simulink model "ModelEquationsDOF4"  (R2022b)
settings: Solver=ode4  StartTime=0.0  StopTime=100  FixedStep=10^-3  RelTol=1e-3
values from neighbouring files (symbols this model uses):
  C1 = 310    [ModelFixedParamDOF4.m]
  C2 = 200    [ModelFixedParamDOF4.m]
  C3 = 9091    [ModelFixedParamDOF4.m]
  C4 = 330    [ModelFixedParamDOF4.m]
  C5 = 2475    [ModelFixedParamDOF4.m]
  Cs = 74518    [OptimizedParamDOF3.m]    (also in OptimizedParamDOF4.m = 900)
  Cse = 150    [ModelFixedParamDOF4.m]
  Ct = 850    [ModelFixedParamDOF3.m]    (also in ModelFixedParamDOF4.m)
  K1 = 166990    [ModelFixedParamDOF4.m]
  K2 = 10000    [ModelFixedParamDOF4.m]
  K3 = 144000    [ModelFixedParamDOF4.m]
  K4 = 20000    [ModelFixedParamDOF4.m]
  K5 = 49340    [ModelFixedParamDOF4.m]
  Ks = 106826    [OptimizedParamDOF3.m]    (also in OptimizedParamDOF4.m = 10039)
  Kse = 15000    [ModelFixedParamDOF4.m]
  Kt = 150000    [ModelFixedParamDOF3.m]    (also in ModelFixedParamDOF4.m)
  m1 = 417    [ModelFixedParamDOF4.m]    (also in ModelFixedParamDOF5.m = 40)
  m2 = 15    [ModelFixedParamDOF4.m]    (also in ModelFixedParamDOF5.m = 35.5)
  m3 = 55    [ModelFixedParamDOF4.m]
  m4 = 36    [ModelFixedParamDOF4.m]
  mb = 250    [ModelFixedParamDOF4.m]
  mse = 35    [ModelFixedParamDOF4.m]
  mw = 25    [ModelFixedParamDOF4.m]
  road_front_wheel = M.'    [LoadRoadScript.m]
settings Model: Creator=Ade  LastModifiedBy=andre
settings SolverCC: AlgebraicLoopSolver=TrustRegion
settings DataIOCC: ReturnWorkspaceOutputs=off
settings DebuggingCC: UnconnectedInputMsg=warning  UnconnectedOutputMsg=warning  UnconnectedLineMsg=warning  SFMachineParentedDataDiag=warning  ArithmeticOperatorsInVariantConditions=warning
settings ModelReferenceCC: EnableRefExpFcnMdlSchedulingChecks=on
settings SFSimCC: SimUseLocalCustomCode=off  CustomCodeUndefinedFunction=UseInterfaceOnly
settings RTWCC: RTWUseLocalCustomCode=off  DLArmComputeVersion=19.05

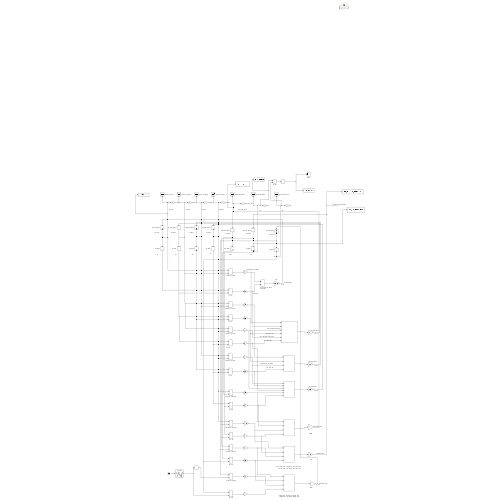
[thumbnail: Simulink's stored preview of the top-level diagram]
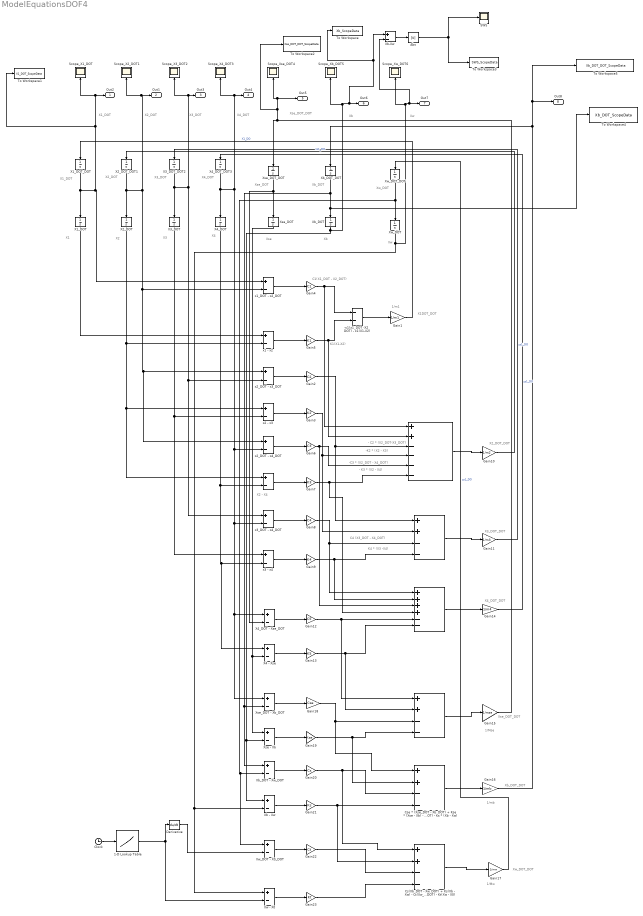
== system ModelEquationsDOF4 ==
  note: 1/Mw
  note: X4_DOT_DOT
  note: X3_DOT_DOT
  note: C4 (X3_DOT - X4_DOT)
  note: K4 * (X3 -X4)
  note: X2 - X4
  note: X2_DOT_DOT
  note: - K3 * (X2 - X4)
  note: -C3 * (X2_DOT - X4_DOT)
  note: K1(X1-X2)
  note: C1(X1_DOT - X2_DOT)
  note: 1/m1
  note: X3
  note: X4
  note: X2
  note: X1_DOT
  note: X1DOT_DOT
  note: X2_DOT
  note: X1
  note: X3_DOT
  note: X4_DOT
  note: -K2 * (X2 - X3)
  note: - C2 * (X2_DOT-X3_DOT)
  note: Xse_DOT
  note: Xse
  note: Xb
  note: Xb_DOT
  note: Xw
  note: Xw_DOT
  note: Xse_DOT_DOT
  note: Xw_DOT_DOT
  note: Xb_DOT_DOT
  note: 1/mb
  note: 1/Mse
  note: X1_DOT
  note: X2_DOT
  note: X3_DOT
  note: X4_DOT
  note: Xse_DOT_DOT
  note: Xb
  note: Xw
  " " : Sum  Inputs=+-
  "      " : Sum  Inputs=++----
  " " : Sum  Inputs=++--
  " " : Sum  Inputs=++++--
  " " : Sum  Inputs=++--
  " Cs(Xb_DOT - Xw_DOT) + Ks(Xb - Xw) - Ct(Xw_DOT - X0_DOT) - Kt(Xw - X0)" : Sum  Inputs=++--
  " Cse * (Xse_DOT - Xb_DOT) + Kse * (Xse - Xb) - Cs * (Xb_DOT - Xw_DOT) - Ks * (Xb - Xw)" : Sum  Inputs=++--
  "                    -c1(x1_DOT -X2_DOT) - k1(X1-X2)" : Sum  Inputs=--
  1-D Lookup Table : Lookup_n-D  NumberOfTableDimensions=1  LookupTableObject=road_front_wheel  BreakpointsForDimension1=[1:100]  Table=road_front_wheel  InternalRulePriority=Speed  RndMeth=Simplest
  Abs : Abs  SaturateOnIntegerOverflow=off
  Clock : Clock
  Derivative : Derivative
  Gain1 : Gain  Gain=1/m1
  Gain10 : Gain  Gain=1/m2
  Gain11 : Gain  Gain=1/m3
  Gain12 : Gain  Gain=C5
  Gain13 : Gain  Gain=K5
  Gain14 : Gain  Gain=1/m4
  Gain15 : Gain  Gain=1/mse
  Gain16 : Gain  Gain=1/mb
  Gain17 : Gain  Gain=1/mw
  Gain18 : Gain  Gain=Cse
  Gain19 : Gain  Gain=Kse
  Gain2 : Gain  Gain=C2
  Gain20 : Gain  Gain=Cs
  Gain21 : Gain  Gain=Ks
  Gain22 : Gain  Gain=Ct
  Gain23 : Gain  Gain=Kt
  Gain3 : Gain  Gain=K2
  Gain4 : Gain  Gain=C1
  Gain5 : Gain  Gain=K1
  Gain6 : Gain  Gain=C3
  Gain7 : Gain  Gain=K3
  Gain8 : Gain  Gain=C4
  Gain9 : Gain  Gain=K4
  SWS : Scope
  Scope_X1_DOT : Scope
  Scope_X2_DOT1 : Scope
  Scope_X3_DOT2 : Scope
  Scope_X4_DOT3 : Scope
  Scope_Xb_DOT5 : Scope
  Scope_Xse_DOT4 : Scope
  Scope_Xw_DOT6 : Scope
  To Workspace : ToWorkspace  VariableName=Xb_ScopeData  SaveFormat=Structure With Time  SampleTime=-1
  To Workspace1 : ToWorkspace  VariableName=X1_DOT_ScopeData  SaveFormat=Structure With Time  SampleTime=-1
  To Workspace2 : ToWorkspace  VariableName=Xse_DOT_DOT_ScopeData  SaveFormat=Structure With Time  SampleTime=-1
  To Workspace3 : ToWorkspace  VariableName=SWS_ScopeData  SaveFormat=Structure With Time  SampleTime=-1
  To Workspace4 : ToWorkspace  VariableName=Xb_DOT_ScopeData  SaveFormat=Structure With Time  SampleTime=-1
  To Workspace5 : ToWorkspace  VariableName=Xb_DOT_DOT_ScopeData  SaveFormat=Structure With Time  SampleTime=-1
  X1_DOT : Integrator
  X1_DOT_DOT : Integrator
  X2_DOT : Integrator
  X2_DOT_DOT1 : Integrator
  X3_DOT : Integrator
  X3_DOT_DOT2 : Integrator
  X4 - Xse : Sum  Inputs=+-
  X4_DOT : Integrator
  X4_DOT - Xse_DOT : Sum  Inputs=+-
  X4_DOT_DOT3 : Integrator
  Xb - Xw : Sum  Inputs=+-
  Xb-Xw : Sum  Inputs=+-
  Xb_DOT : Integrator
  Xb_DOT - Xw_DOT : Sum  Inputs=+-
  Xb_DOT_DOT : Integrator
  Xse - Xb : Sum  Inputs=+-
  Xse_DOT : Integrator
  Xse_DOT - Xb_DOT : Sum  Inputs=+-
  Xse_DOT_DOT : Integrator
  Xw - X0 : Sum  Inputs=+-
  "Xw_DOT " : Integrator
  "Xw_DOT - X0_DOT " : Sum  Inputs=+-
  "Xw_DOT_DOT " : Integrator
  x1 - x2 : Sum  Inputs=+-
  x1_DOT - x2_DOT : Sum  Inputs=+-
  x2 - x3 : Sum  Inputs=+-
  x2_DOT - x3_DOT : Sum  Inputs=+-
  x2_DOT - x4_DOT : Sum  Inputs=+-
  x3 - x4 : Sum  Inputs=+-
  x3_DOT - x4_DOT : Sum  Inputs=+-
  Out2 : Outport  SignalName=X1_DOT  VectorParamsAs1DForOutWhenUnconnected=off
  Out1 : Outport  Port=2  SignalName=X2_DOT  VectorParamsAs1DForOutWhenUnconnected=off
  Out3 : Outport  Port=3  SignalName=X3_DOT  VectorParamsAs1DForOutWhenUnconnected=off
  Out4 : Outport  Port=4  SignalName=X4_DOT  VectorParamsAs1DForOutWhenUnconnected=off
  Out5 : Outport  Port=5  SignalName=Xse_DOT_DOT  VectorParamsAs1DForOutWhenUnconnected=off
  Out6 : Outport  Port=6  SignalName=Xb  VectorParamsAs1DForOutWhenUnconnected=off
  Out7 : Outport  Port=7  SignalName=Xw  VectorParamsAs1DForOutWhenUnconnected=off
  Out8 : Outport  Port=8  SignalName=Xb_DOT_DOT  VectorParamsAs1DForOutWhenUnconnected=off
  wires:
  X3_DOT_DOT2/1 -> Scope_X3_DOT2/1, Out3/1, x2_DOT - x3_DOT/2, x3_DOT - x4_DOT/1, X3_DOT/1
  X4_DOT_DOT3/1 -> Scope_X4_DOT3/1, Out4/1, Xse_DOT - Xb_DOT/1, X4_DOT - Xse_DOT/1, x3_DOT - x4_DOT/2, x2_DOT - x4_DOT/2, X4_DOT/1
  X3_DOT/1 -> x3 - x4/1, x2 - x3/2
  Gain4/1 -> "      "/1, "                    -c1(x1_DOT -X2_DOT) - k1(X1-X2)"/1
  X1_DOT_DOT/1 -> To Workspace1/1, Out2/1, Scope_X1_DOT/1, x1_DOT - x2_DOT/1, X1_DOT/1
  X4_DOT/1 -> X4 - Xse/1, x3 - x4/2, " "/2
  Gain5/1 -> "      "/2, "                    -c1(x1_DOT -X2_DOT) - k1(X1-X2)"/2
  x1_DOT - x2_DOT/1 -> Gain4/1
  x1 - x2/1 -> Gain5/1
  X2_DOT/1 -> " "/1, x2 - x3/1, x1 - x2/2
  "                    -c1(x1_DOT -X2_DOT) - k1(X1-X2)"/1 -> Gain1/1
  X1_DOT/1 -> x1 - x2/1
  x2 - x3/1 -> Gain3/1
  x2_DOT - x3_DOT/1 -> Gain2/1
  x2_DOT - x4_DOT/1 -> Gain6/1
  " "/1 -> Gain7/1
  x3 - x4/1 -> Gain9/1
  x3_DOT - x4_DOT/1 -> Gain8/1
  Gain2/1 -> " "/1, "      "/3
  Gain3/1 -> " "/2, "      "/4
  Gain6/1 -> " "/3, "      "/5
  Gain7/1 -> " "/4, "      "/6
  "      "/1 -> Gain10/1
  Gain8/1 -> " "/1, " "/3
  Gain9/1 -> " "/2, " "/4
  " "/1 -> Gain11/1
  " "/1 -> Gain14/1
  X4_DOT - Xse_DOT/1 -> Gain12/1
  X4 - Xse/1 -> Gain13/1
  Gain12/1 -> " "/1, " "/5
  Gain13/1 -> " "/2, " "/6
  Xse_DOT_DOT/1 -> X4_DOT - Xse_DOT/2, Xse_DOT/1
  Xse_DOT/1 -> Xse - Xb/1, X4 - Xse/2
  Xb_DOT/1 -> Scope_Xb_DOT5/1, To Workspace/1, Xb-Xw/1, Out6/1, Xb - Xw/1, Xse - Xb/2
  Xb_DOT_DOT/1 -> Xb_DOT - Xw_DOT/1, Xse_DOT - Xb_DOT/2, Xb_DOT/1, To Workspace4/1
  " "/1 -> Gain15/1
  " Cse * (Xse_DOT - Xb_DOT) + Kse * (Xse - Xb) - Cs * (Xb_DOT - Xw_DOT) - Ks * (Xb - Xw)"/1 -> Gain16/1
  " Cs(Xb_DOT - Xw_DOT) + Ks(Xb - Xw) - Ct(Xw_DOT - X0_DOT) - Kt(Xw - X0)"/1 -> Gain17/1
  Xse - Xb/1 -> Gain19/1
  Xse_DOT - Xb_DOT/1 -> Gain18/1
  Xb - Xw/1 -> Gain21/1
  Xb_DOT - Xw_DOT/1 -> Gain20/1
  Xw - X0/1 -> Gain23/1
  "Xw_DOT - X0_DOT "/1 -> Gain22/1
  Gain23/1 -> " Cs(Xb_DOT - Xw_DOT) + Ks(Xb - Xw) - Ct(Xw_DOT - X0_DOT) - Kt(Xw - X0)"/4
  Gain22/1 -> " Cs(Xb_DOT - Xw_DOT) + Ks(Xb - Xw) - Ct(Xw_DOT - X0_DOT) - Kt(Xw - X0)"/3
  Gain21/1 -> " Cs(Xb_DOT - Xw_DOT) + Ks(Xb - Xw) - Ct(Xw_DOT - X0_DOT) - Kt(Xw - X0)"/2, " Cse * (Xse_DOT - Xb_DOT) + Kse * (Xse - Xb) - Cs * (Xb_DOT - Xw_DOT) - Ks * (Xb - Xw)"/4
  Gain20/1 -> " Cs(Xb_DOT - Xw_DOT) + Ks(Xb - Xw) - Ct(Xw_DOT - X0_DOT) - Kt(Xw - X0)"/1, " Cse * (Xse_DOT - Xb_DOT) + Kse * (Xse - Xb) - Cs * (Xb_DOT - Xw_DOT) - Ks * (Xb - Xw)"/3
  Gain18/1 -> " Cse * (Xse_DOT - Xb_DOT) + Kse * (Xse - Xb) - Cs * (Xb_DOT - Xw_DOT) - Ks * (Xb - Xw)"/1, " "/3
  Gain19/1 -> " Cse * (Xse_DOT - Xb_DOT) + Kse * (Xse - Xb) - Cs * (Xb_DOT - Xw_DOT) - Ks * (Xb - Xw)"/2, " "/4
  "Xw_DOT_DOT "/1 -> "Xw_DOT - X0_DOT "/1, Xb_DOT - Xw_DOT/2, "Xw_DOT "/1
  Gain1/1 -> X1_DOT_DOT/1  "X1_DO"
  Gain10/1 -> X2_DOT_DOT1/1  "zs1_DO"
  Gain11/1 -> X3_DOT_DOT2/1  "zs1_DO"
  Gain14/1 -> X4_DOT_DOT3/1  "zs1_DO"
  Gain16/1 -> Out8/1, To Workspace5/1, Xb_DOT_DOT/1
  Gain17/1 -> "Xw_DOT_DOT "/1  "zs1_DO"
  X2_DOT_DOT1/1 -> Out1/1, Scope_X2_DOT1/1, x2_DOT - x4_DOT/1, x2_DOT - x3_DOT/1, x1_DOT - x2_DOT/2, X2_DOT/1
  1-D Lookup Table/1 -> Derivative/1, Xw - X0/2
  "Xw_DOT "/1 -> Scope_Xw_DOT6/1, Xb-Xw/2, Out7/1, Xw - X0/1, Xb - Xw/2
  Gain15/1 -> To Workspace2/1, Scope_Xse_DOT4/1, Out5/1, Xse_DOT_DOT/1
  Derivative/1 -> "Xw_DOT - X0_DOT "/2
  Clock/1 -> 1-D Lookup Table/1
  Xb-Xw/1 -> Abs/1
  Abs/1 -> SWS/1, To Workspace3/1
